simulink model "ACASXU_Simulink"  (R2026a)
settings: Solver=FixedStepDiscrete  FixedStep=0.01
values from neighbouring files (symbols this model uses):
  quantizedNet = quantize(qObj)    [run_acasxu_pipeline.m]
libraries: dlconvfclib x7, dlactivationlib x6
settings Model: Creator=arkadiyturevskiy  LastModifiedBy=arkadiyturevskiy
settings RTWCC: SystemTargetFile=ert.tlc  GenCodeOnly=on  Description=Embedded Coder
settings ERTTargetCC: GenerateSampleERTMain=on

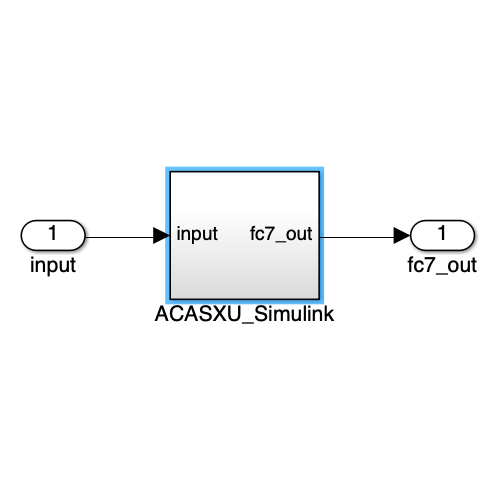
[thumbnail: Simulink's stored preview of the top-level diagram]
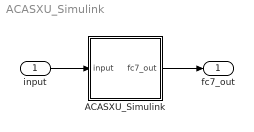
== system ACASXU_Simulink ==
  input : Inport  PortDimensions=[5]
  ACASXU_Simulink : Subsystem
  fc7_out : Outport
  wires:
  ACASXU_Simulink/1(fc7_out) -> fc7_out/1
  input/1 -> ACASXU_Simulink/1(input)

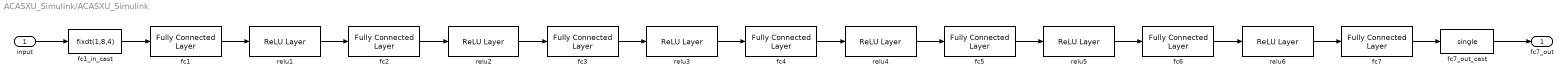
== system ACASXU_Simulink/ACASXU_Simulink ==
  input : Inport  PortDimensions=[5]
  fc1 : dlconvfclib/Fully Connected Layer  Layer=quantizedNet.Layers(2)  OutMin=[]  OutMax=[]  OutDataTypeStr=fixdt(1,8,5)  RndMeth=Nearest  SaturateOnIntegerOverflow=on  WeightsDataTypeStr=fixdt(1,8,7)  WeightsMin=[]  WeightsMax=[]  BiasDataTypeStr=fixdt(1,32,11)  BiasMin=[]  BiasMax=[]  AccumDataTypeStr=fixdt(1,32,11)  AccumMin=[]  AccumMax=[]  InternalRndMeth=Nearest  InternalSaturateOnIntegerOverflow=off  SampleTime=-1
      settings: DataFormat=C
  fc1_in_cast : DataTypeConversion  OutDataTypeStr=fixdt(1,8,4)  RndMeth=Nearest
  fc2 : dlconvfclib/Fully Connected Layer  Layer=quantizedNet.Layers(4)  OutMin=[]  OutMax=[]  OutDataTypeStr=fixdt(1,8,5)  RndMeth=Nearest  SaturateOnIntegerOverflow=on  WeightsDataTypeStr=fixdt(1,8,3)  WeightsMin=[]  WeightsMax=[]  BiasDataTypeStr=fixdt(1,32,8)  BiasMin=[]  BiasMax=[]  AccumDataTypeStr=fixdt(1,32,8)  AccumMin=[]  AccumMax=[]  InternalRndMeth=Nearest  InternalSaturateOnIntegerOverflow=off  SampleTime=-1
      settings: DataFormat=C
  fc3 : dlconvfclib/Fully Connected Layer  Layer=quantizedNet.Layers(6)  OutMin=[]  OutMax=[]  OutDataTypeStr=fixdt(1,8,4)  RndMeth=Nearest  SaturateOnIntegerOverflow=on  WeightsDataTypeStr=fixdt(1,8,3)  WeightsMin=[]  WeightsMax=[]  BiasDataTypeStr=fixdt(1,32,8)  BiasMin=[]  BiasMax=[]  AccumDataTypeStr=fixdt(1,32,8)  AccumMin=[]  AccumMax=[]  InternalRndMeth=Nearest  InternalSaturateOnIntegerOverflow=off  SampleTime=-1
      settings: DataFormat=C
  fc4 : dlconvfclib/Fully Connected Layer  Layer=quantizedNet.Layers(8)  OutMin=[]  OutMax=[]  OutDataTypeStr=fixdt(1,8,1)  RndMeth=Nearest  SaturateOnIntegerOverflow=on  WeightsDataTypeStr=fixdt(1,8,3)  WeightsMin=[]  WeightsMax=[]  BiasDataTypeStr=fixdt(1,32,7)  BiasMin=[]  BiasMax=[]  AccumDataTypeStr=fixdt(1,32,7)  AccumMin=[]  AccumMax=[]  InternalRndMeth=Nearest  InternalSaturateOnIntegerOverflow=off  SampleTime=-1
      settings: DataFormat=C
  fc5 : dlconvfclib/Fully Connected Layer  Layer=quantizedNet.Layers(10)  OutMin=[]  OutMax=[]  OutDataTypeStr=fixdt(1,8,1)  RndMeth=Nearest  SaturateOnIntegerOverflow=on  WeightsDataTypeStr=fixdt(1,8,3)  WeightsMin=[]  WeightsMax=[]  BiasDataTypeStr=fixdt(1,32,4)  BiasMin=[]  BiasMax=[]  AccumDataTypeStr=fixdt(1,32,4)  AccumMin=[]  AccumMax=[]  InternalRndMeth=Nearest  InternalSaturateOnIntegerOverflow=off  SampleTime=-1
      settings: DataFormat=C
  fc6 : dlconvfclib/Fully Connected Layer  Layer=quantizedNet.Layers(12)  OutMin=[]  OutMax=[]  OutDataTypeStr=fixdt(1,8,3)  RndMeth=Nearest  SaturateOnIntegerOverflow=on  WeightsDataTypeStr=fixdt(1,8,2)  WeightsMin=[]  WeightsMax=[]  BiasDataTypeStr=fixdt(1,32,3)  BiasMin=[]  BiasMax=[]  AccumDataTypeStr=fixdt(1,32,3)  AccumMin=[]  AccumMax=[]  InternalRndMeth=Nearest  InternalSaturateOnIntegerOverflow=off  SampleTime=-1
      settings: DataFormat=C
  fc7 : dlconvfclib/Fully Connected Layer  Layer=quantizedNet.Layers(14)  OutMin=[]  OutMax=[]  OutDataTypeStr=fixdt(1,32,2)  RndMeth=Nearest  WeightsDataTypeStr=fixdt(1,8,-1)  WeightsMin=[]  WeightsMax=[]  BiasDataTypeStr=fixdt(1,32,2)  BiasMin=[]  BiasMax=[]  AccumDataTypeStr=fixdt(1,32,2)  AccumMin=[]  AccumMax=[]  InternalRndMeth=Nearest  InternalSaturateOnIntegerOverflow=off  SampleTime=-1
      settings: DataFormat=C
  fc7_out_cast : DataTypeConversion  OutDataTypeStr=single  SaturateOnIntegerOverflow=off  RndMeth=Floor
  relu1 : dlactivationlib/ReLU Layer  OutMin=[]  OutMax=[]  OutDataTypeStr=fixdt(1,8,5)  SampleTime=-1
  relu2 : dlactivationlib/ReLU Layer  OutMin=[]  OutMax=[]  OutDataTypeStr=fixdt(1,8,5)  SampleTime=-1
  relu3 : dlactivationlib/ReLU Layer  OutMin=[]  OutMax=[]  OutDataTypeStr=fixdt(1,8,4)  SampleTime=-1
  relu4 : dlactivationlib/ReLU Layer  OutMin=[]  OutMax=[]  OutDataTypeStr=fixdt(1,8,1)  SampleTime=-1
  relu5 : dlactivationlib/ReLU Layer  OutMin=[]  OutMax=[]  OutDataTypeStr=fixdt(1,8,1)  SampleTime=-1
  relu6 : dlactivationlib/ReLU Layer  OutMin=[]  OutMax=[]  OutDataTypeStr=fixdt(1,8,3)  SampleTime=-1
  fc7_out : Outport
  wires:
  relu1/1 -> fc2/1
  fc1_in_cast/1 -> fc1/1
  relu5/1 -> fc6/1
  fc6/1 -> relu6/1
  fc7/1 -> fc7_out_cast/1
  fc4/1 -> relu4/1
  relu3/1 -> fc4/1
  relu4/1 -> fc5/1
  fc5/1 -> relu5/1
  relu2/1 -> fc3/1
  fc7_out_cast/1 -> fc7_out/1
  fc1/1 -> relu1/1
  relu6/1 -> fc7/1
  fc2/1 -> relu2/1
  input/1 -> fc1_in_cast/1
  fc3/1 -> relu3/1
